simulink model "Controlador_ON_OFF_Def"  (R2026a)
settings: Solver=VariableStepAuto
settings Model: Creator=Nehir RT  LastModifiedBy=Nehir RT

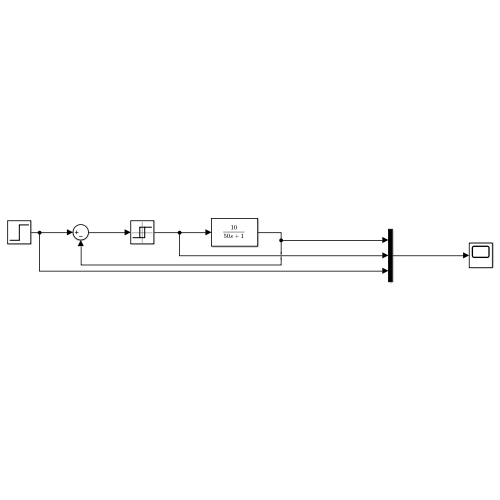
[thumbnail: Simulink's stored preview of the top-level diagram]
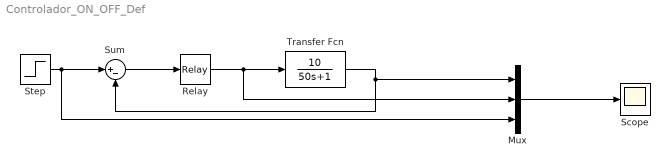
== system Controlador_ON_OFF_Def ==
  Mux : Mux  Inputs=3
  Relay : Relay  OnSwitchValue=0.5  OffSwitchValue=-0.5  OnOutputValue=100
  Scope : Scope
      settings: ActiveDisplayYMinimum=-12.089408995211654  ActiveDisplayYMaximum=14.712503817288344
  Step : Step  FinalValue=80  SampleTime=0
  Sum : Sum  Inputs=|+-
  Transfer Fcn : TransferFcn  Numerator=[10]  Denominator=[50 1]
  wires:
  Step/1 -> Mux/3, Sum/1
  Relay/1 -> Mux/2, Transfer Fcn/1
  Sum/1 -> Relay/1
  Transfer Fcn/1 -> Sum/2, Mux/1
  Mux/1 -> Scope/1
